simulink model "ClosedLoopSystem_PID_Exp_python_block"  (R2025b)
settings: Solver=FixedStepAuto  StartTime=0.0  StopTime=100  RelTol=1e-3  EnableMultiTasking=on
undefined symbols (not defined in the file): ref_angle, tf_raspi, ts_raspi
libraries: simulink_extras x2, simulink x1
settings Model: DataDictionary=sys_PID_data.sldd  ExtModeTrigDuration=2  Creator=tshintai  LastModifiedBy=abuj
settings SolverCC: PositivePriorityOrder=on
settings OptimizationCC: EnhancedBackFolding=on  PassReuseOutputArgsAs=Individual arguments  ZeroExternalMemoryAtStartup=off  ZeroInternalMemoryAtStartup=off  MaxStackSize=200000  OptimizeBlockOrder=speed  DifferentSizesBufferReuse=on  OptimizationCustomize=off  EfficientTunableParamExpr=on
settings DebuggingCC: ParameterTunabilityLossMsg=error  UnconnectedInputMsg=warning  UnconnectedOutputMsg=warning  UnconnectedLineMsg=warning
settings HardwareCC: ProdBitPerPointer=32.0  ProdBitPerSizeT=32.0  ProdBitPerPtrDiffT=32.0  ProdLargestAtomicInteger=Long  ProdLargestAtomicFloat=Double  ProdWordSize=32.0  ProdLongLongMode=on  ProdHWDeviceType=ARM Compatible->ARM Cortex-A (32-bit)
settings ModelReferenceCC: EnableRefExpFcnMdlSchedulingChecks=on
settings RTWCC: SystemTargetFile=ert.tlc  HardwareBoard=Raspberry Pi  TLCOptions="-aInlineSetEventsForThisBaseRateFcn=TLC_FALSE -aSuppressMultiTaskScheduler=TLC_FALSE  -aRateBasedStepFcn=0"  TemplateMakefile=ert_default_tmf  Toolchain=GNU GCC Embedded Linux  BuildConfiguration=Faster Runs  GPUComputeCapability=3.5  DLArmComputeVersion=19.05  Description=Embedded Coder
settings CodeAppCC: ForceParamTrailComments=on  IgnoreCustomStorageClasses=off  OperatorAnnotations=on  SimulinkDataObjDesc=on  SFDataObjDesc=on  InsertBlockDesc=on
settings ERTTargetCC: ExtModeTransport=2.0  ExtModeStaticAlloc=on  ExtModeMexFile=ext_xcp  ExtModeIntrfLevel=Level2 - Open  InlinedParameterPlacement=Hierarchical  DynamicArrayContainerType=coder::array  SupportVariableSizeSignals=on

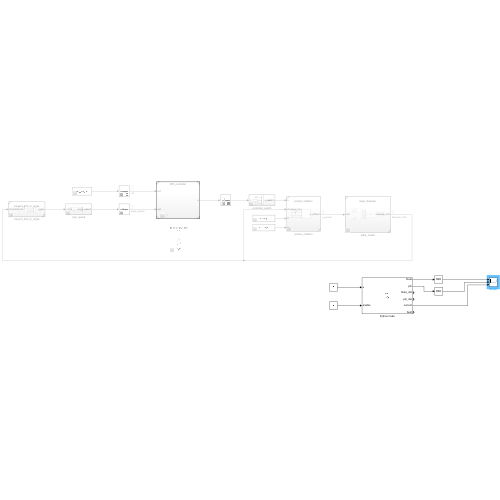
[thumbnail: Simulink's stored preview of the top-level diagram]
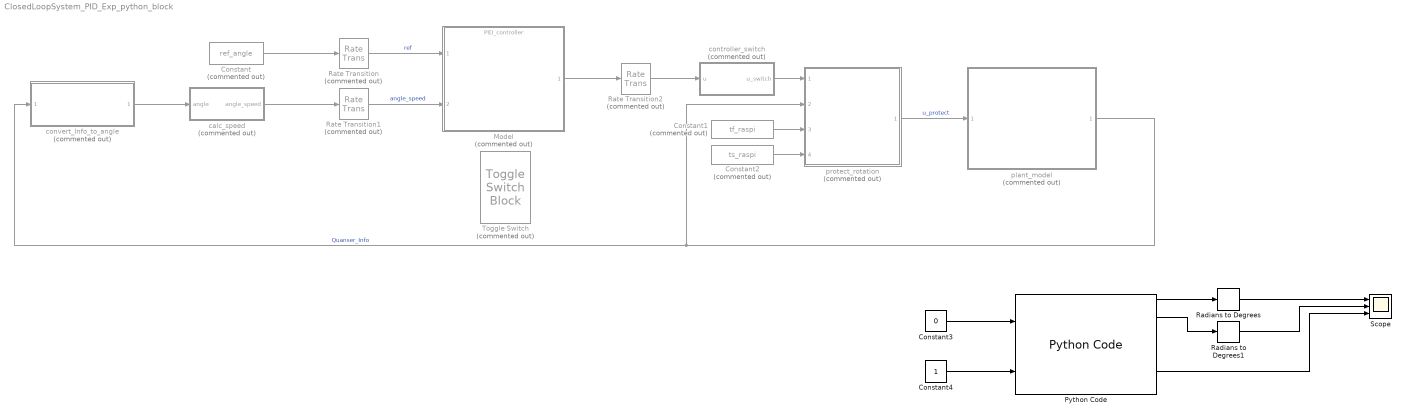
== system ClosedLoopSystem_PID_Exp_python_block ==
  Constant : Constant  Commented=on  Value=ref_angle
  Constant1 : Constant  Commented=on  Value=tf_raspi
  Constant2 : Constant  Commented=on  Value=ts_raspi
  Constant3 : Constant  Value=0  OutDataTypeStr=double
  Constant4 : Constant  OutDataTypeStr=boolean
  Model : ModelReference  Commented=on  ModelNameDialog=PID_controller.slx  SimulationMode=Normal  ModelReferenceVersion=2.2
  Python Code : PythonCode  InitializeConditionsCode=|  OutputCode=|  TerminateCode=|  SampleTime=0.005
      InitializeConditionsCode=|
      | from rl_qube.simulink.qube3_block import start
      | 
      | start(frequency=200, vlimit=2.0)
      OutputCode=|
      | from rl_qube.simulink.qube3_block import step
      | #import time
      | #time.sleep(3) # Sleep for 3 seconds
      | 
      | theta, phi, theta_dot, phi_dot, current, fault = step(u, enable)
      TerminateCode=|
      | from rl_qube.simulink.qube3_block import stop
      | 
      | stop()
  Radians to Degrees : simulink_extras/Transformations/Radians to Degrees
  Radians to Degrees1 : simulink_extras/Transformations/Radians to Degrees
  Rate Transition : RateTransition  Commented=on  OutPortSampleTime=ts_PID
  Rate Transition1 : RateTransition  Commented=on  OutPortSampleTime=ts_PID
  Rate Transition2 : RateTransition  Commented=on  OutPortSampleTime=ts_raspi
  Scope : Scope  NumInputPorts=3
      settings: ActiveDisplayYMinimum=-174.0234375  ActiveDisplayYMaximum=165.23437499999997
  Toggle Switch : ToggleSwitchBlock  Commented=on
  calc_speed : Subsystem  Commented=on
  controller_switch : Subsystem  Commented=on
  convert_Info_to_angle : Subsystem  Commented=on  ReferencedSubsystem=convert_Info_to_angle
  plant_model : Subsystem  Commented=on  ReferencedSubsystem=raspi_Quanser
  protect_rotation : Subsystem  Commented=on  ReferencedSubsystem=protect_rotation
  wires:
  Constant1/1 -> protect_rotation/3
  protect_rotation/1 -> plant_model/1  "u_protect"
  Constant2/1 -> protect_rotation/4
  Rate Transition2/1 -> controller_switch/1(u)
  plant_model/1 -> protect_rotation/2, convert_Info_to_angle/1  "Quanser_Info"
  Model/1 -> Rate Transition2/1
  Rate Transition/1 -> Model/1  "ref"
  Rate Transition1/1 -> Model/2  "angle_speed"
  Constant/1 -> Rate Transition/1
  convert_Info_to_angle/1 -> calc_speed/1(angle)
  calc_speed/1(angle_speed) -> Rate Transition1/1
  controller_switch/1(u_switch) -> protect_rotation/1
  Constant3/1 -> Python Code/1
  Constant4/1 -> Python Code/2
  Python Code/1 -> Radians to Degrees/1
  Python Code/2 -> Radians to Degrees1/1
  Python Code/5 -> Scope/3
  Radians to Degrees/1 -> Scope/1
  Radians to Degrees1/1 -> Scope/2

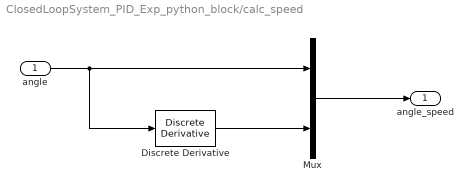
== system ClosedLoopSystem_PID_Exp_python_block/calc_speed ==
  angle : Inport
  Discrete Derivative : simulink/Discrete/Discrete Derivative  gainval=1.0  ICPrevScaledInput=0.0  OutMin=[]  OutMax=[]  OutDataType=fixdt(1, 16)  OutScaling=2^-10  DoSatur=off
  Mux : Mux  Inputs=2
  angle_speed : Outport
  wires:
  Mux/1 -> angle_speed/1
  angle/1 -> Discrete Derivative/1, Mux/1
  Discrete Derivative/1 -> Mux/2

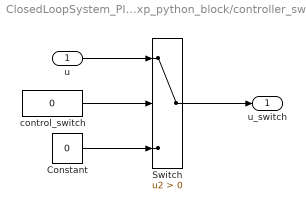
== system ClosedLoopSystem_PID_Exp_python_block/controller_switch ==
  u : Inport
  Constant : Constant  Value=0
  Switch : Switch  Criteria=u2 > Threshold  SaturateOnIntegerOverflow=off  InputSameDT=off
  control_switch : Constant  Value=0  OutDataTypeStr=boolean
  u_switch : Outport
  wires:
  u/1 -> Switch/1
  control_switch/1 -> Switch/2
  Constant/1 -> Switch/3
  Switch/1 -> u_switch/1
